simulink model "lb233_rtlsdr_rx_ppm"  (R2018b)
settings: Solver=VariableStepAuto  StartTime=0.0  StopTime=inf  RelTol=1e-3
undefined symbols (not defined in the file or in its folder): designMultirateFIR
libraries: dspmlti4 x1, dspstat3 x1, sdrrlib x1
settings Model: Creator=Григорий Фокин  LastModifiedBy=Григорий Фокин
settings SFSimCC: SimUseLocalCustomCode=off
settings RTWCC: RTWUseLocalCustomCode=off
settings CodeAppCC: StateflowObjectComments=on

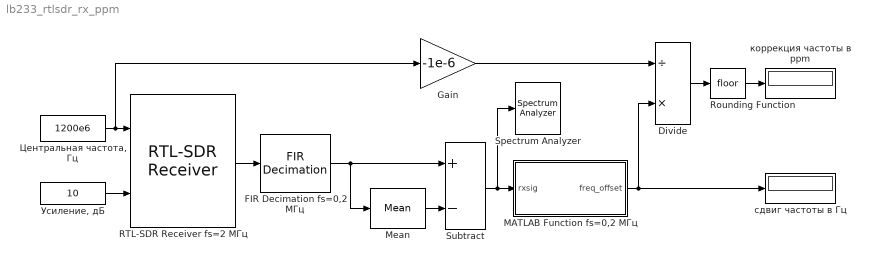
== system lb233_rtlsdr_rx_ppm ==
  Divide : Product  Inputs=/*
  FIR Decimation fs=0,2 МГц : dspmlti4/FIR Decimation  FilterSource=Auto  h=designMultirateFIR(1,2)  D=10  filtStruct=Direct form  FilterObject=FDECIM  InputProcessing=Columns as channels (frame based)  framing=Allow multirate processing  inputOffset=0  outputBufInitCond=0  roundingMode=Floor  overflowMode=off  firstCoeffDataTypeStr=Inherit: Same word length as input  firstCoeffMin=[]  firstCoeffMax=[]  firstCoeffLastDataTypeStr=Inherit: Same word length as input  outputDataTypeStr=Inherit: Same as accumulator  outputMin=[]  outputMax=[]  outputLastDataTypeStr=Inherit: Same as accumulator
  Gain : Gain  Gain=-1e-6
  MATLAB Function fs=0,2 МГц : MATLAB Function  TreatAsAtomicUnit=on
  Mean : dspstat3/Mean  run=off  InputProcessing=Columns as channels (frame based)  reset_popup=None  directionMode=Each column  dimension=1  roiEnable=off  roiType=Rectangles  roiPortion=Entire ROI  roiOutput=Individual statistics for each ROI  roiFlag=off  roundingMode=Floor  overflowMode=off  outputDataTypeStr=Inherit: Same as accumulator  outputMin=[]  outputMax=[]  outputLastDataTypeStr=Inherit: Same as accumulator
  RTL-SDR Receiver fs=2 МГц : sdrrlib/RTL-SDR Receiver  IPAddress=0  CenterFrequencySource=Input port  CenterFrequency=102.5e6  GainSource=Input port  Gain=0  ADCRate=2e6  FrequencyCorrection=89  LostSamplesOutputPort=off  LatencyOutputPort=off  OutputDataType=single  FrameLength=4096  EnableBurstMode=off  NumFramesInBurst=20  sobjType=sdrr.internal.SDRRTLReceiverSL  dataUDPPort=-1  ctrlUDPPort=-1  subDeviceList=nosubdev  sdrBlockType=SDRBlockTypeSLT.SDRRxBlock  requester=UNUSED_BY_SFCN  sdrExecutionMode=SDRExecutionModeSLT.ExecModeHW  BypassUserLogic=off  DecimatorSelect=DDC decimator  SourceSelect=RF data  SineAmplitude=16000  EnableInternalClock=off  BypassIQBalance=off  IFBandwidth=40e6  ADCRateSource=Dialog  IntermediateFrequency=0  DecimationFactorSource=Dialog  DecimationFactor=512  RFFrequencyIsTunable=logical(1)  SampleTime=(4096)/(2e6)  IFBandwidthSource=Dialog  SineFrequency=30000  BypassDCBlockingFilter=off  IntermediateFrequencySource=Dialog  IQBalanceCoefficients=64  SkipAllHardwareResetAndInitialization=off  EnableIQCalibrationTable=on  CacheIQCalibrationTable=off  EnableOffsetTuning=off  EnableRTLAGC=off  EnableTestMode=off  EnableTunerAGC=off  FrequencyCorrectionSource=Dialog  NumMLBuffers=128  NumUSBBuffers=16  RTLCrystalFrequency=28800000  TunerCrystalFrequency=28800000
      settings: SourceProductName=Communications System Toolbox Support Package for RTL-SDR Radio  SourceProductBaseCode=RTLSDR
  Rounding Function : Rounding
  Spectrum Analyzer : SpectrumAnalyzer
  Subtract : Sum  Inputs=+-
  "Усиление, дБ" : Constant  Value=10
  "Центральная частота, Гц" : Constant  Value=1200e6
  коррекция частоты в ppm : Display
  сдвиг частоты в Гц : Display
  wires:
  "Усиление, дБ"/1 -> RTL-SDR Receiver fs=2 МГц/2
  "Центральная частота, Гц"/1 -> Gain/1, RTL-SDR Receiver fs=2 МГц/1
  Mean/1 -> Subtract/2
  RTL-SDR Receiver fs=2 МГц/1 -> FIR Decimation fs=0,2 МГц/1
  Subtract/1 -> MATLAB Function fs=0,2 МГц/1(rxsig), Spectrum Analyzer/1
  Gain/1 -> Divide/1
  MATLAB Function fs=0,2 МГц/1(freq_offset) -> сдвиг частоты в Гц/1, Divide/2
  Divide/1 -> Rounding Function/1
  Rounding Function/1 -> коррекция частоты в ppm/1
  FIR Decimation fs=0,2 МГц/1 -> Subtract/1, Mean/1

== matlab function lb233_rtlsdr_rx_ppm/MATLAB Function fs=0,2 МГц ==
  data: rxsig input; freq_offset output
function freq_offset  = freqoffset(rxsig)
% freq_offset - входной сигнал
% freq_offset - сдвиг частот, Гц
nfft = 8192; % размерность БПФ
fs = 0.2e6;  % частота дискретизации входного сигнала, Гц
delta_f = fs/nfft; % БПФ разрешение по частоте // fft bin
% Вычисление БПФ сигнала rxsig: [+ve freqs , -ve freqs]
fft_sig = fft(rxsig,nfft);    
% Преобразование сигнала fft_sig: [-ve freqs , +ve freqs]
fft_sig = fftshift(fft_sig);
% Нахождение индекса максимальной выборки fft_sig
[~, max_idx] = max(fft_sig); 
% Оценка индекса сдвига частот по индексу max_idx: 
% преобразование max_idx для симметрии относительно 0
offset_idx = max_idx-1-nfft/2;   
% Отображение индекса сдвига частот в значение сдвига частот
freq_offset = offset_idx*delta_f; 
end
